simulink subsystem "coeff_bank_multiple_rams"  (R2021b)
settings: Solver=VariableStepAuto  StartTime=0.0  StopTime=10.0  RelTol=1e-3
undefined symbols (not defined in the file): num_rams
libraries: simulink x3, hdlsllib x2
settings Model: Creator=torha  LastModifiedBy=torha
settings SolverCC: AlgebraicLoopSolver=TrustRegion
settings DebuggingCC: SFMachineParentedDataDiag=warning

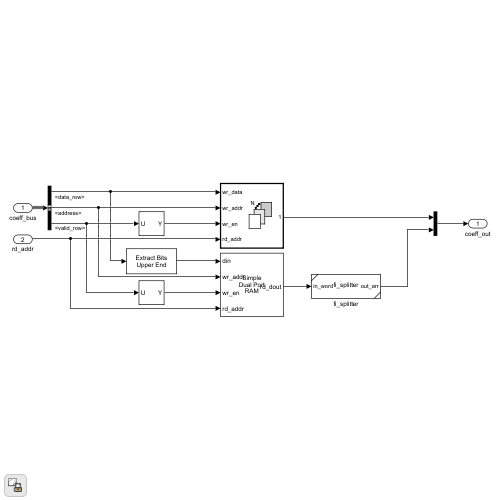
[thumbnail: Simulink's stored preview of the top-level diagram]
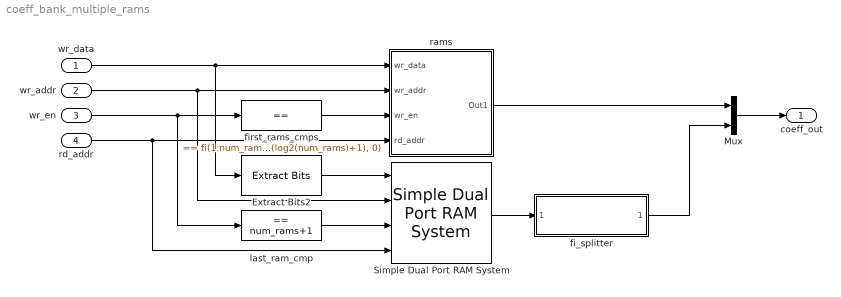
== system coeff_bank_multiple_rams ==
  wr_data : Inport
  wr_addr : Inport  Port=2
  wr_en : Inport  Port=3
  rd_addr : Inport  Port=4
  Extract Bits2 : simulink/Logic and Bit Operations/Extract Bits  bitsToExtract=Range starting with most significant bit  numBits=last_ram_size  bitIdxRange=[0 7]  outScalingMode=Treat bit field as an integer
  Mux : Mux  Inputs=2
  Simple Dual Port RAM System : hdlsllib/HDL RAMs/Simple Dual Port RAM System  RAMType=Simple dual port  WriteOutputValue=New data  RAMInitialValue=0  SimulateUsing=Code generation
      settings: SourceProductBaseCode=SL
  fi_splitter : Subsystem  ReferencedSubsystem=fi_splitter  in_bitwidth=last_ram_size  out_bitwidth=coeff.coeff_bitwidth
  first_rams_cmps : simulink/Logic and Bit Operations/Compare To Constant  relop===  const=fi(1:num_rams, false, floor(log2(num_rams)+1), 0)  OutDataTypeStr=boolean
  last_ram_cmp : simulink/Logic and Bit Operations/Compare To Constant  relop===  const=num_rams+1  OutDataTypeStr=boolean
  rams : Subsystem  TreatAsAtomicUnit=on
  coeff_out : Outport
  wires:
  wr_en/1 -> first_rams_cmps/1, last_ram_cmp/1
  first_rams_cmps/1 -> rams/3(wr_en)
  rams/1(Out1) -> Mux/1
  wr_data/1 -> Extract Bits2/1, rams/1(wr_data)
  wr_addr/1 -> Simple Dual Port RAM System/2, rams/2(wr_addr)
  last_ram_cmp/1 -> Simple Dual Port RAM System/3
  Extract Bits2/1 -> Simple Dual Port RAM System/1
  rd_addr/1 -> rams/4(rd_addr), Simple Dual Port RAM System/4
  Mux/1 -> coeff_out/1
  fi_splitter/1 -> Mux/2
  Simple Dual Port RAM System/1 -> fi_splitter/1

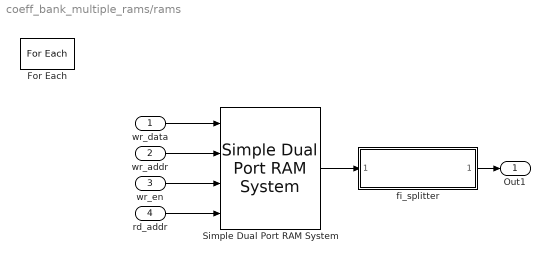
== system coeff_bank_multiple_rams/rams ==
  wr_data : Inport
  wr_addr : Inport  Port=2
  wr_en : Inport  Port=3  Partition=on  PartitionDimension=1  PartitionWidth=1  PartitionOffset=0
  rd_addr : Inport  Port=4
  For Each : ForEach  DisableCoverage=on
  Simple Dual Port RAM System : hdlsllib/HDL RAMs/Simple Dual Port RAM System  RAMType=Simple dual port  WriteOutputValue=New data  RAMInitialValue=0  SimulateUsing=Code generation
      settings: SourceProductBaseCode=SL
  fi_splitter : Subsystem  ReferencedSubsystem=fi_splitter  in_bitwidth=coeff_ram_bitwidth  out_bitwidth=coeff.coeff_bitwidth
  Out1 : Outport  ConcatenationDimension=2
  wires:
  fi_splitter/1 -> Out1/1
  Simple Dual Port RAM System/1 -> fi_splitter/1
  wr_data/1 -> Simple Dual Port RAM System/1
  wr_addr/1 -> Simple Dual Port RAM System/2
  rd_addr/1 -> Simple Dual Port RAM System/4
  wr_en/1 -> Simple Dual Port RAM System/3
